simulink model "Eq_Zeq_circuit"  (R2022b)
settings: Solver=VariableStepAuto  StartTime=0.0  StopTime=10.0  RelTol=1e-3
libraries: nesl_utility x8, fl_lib x7, ee_lib x2
settings Model: Creator=umber  LastModifiedBy=umber

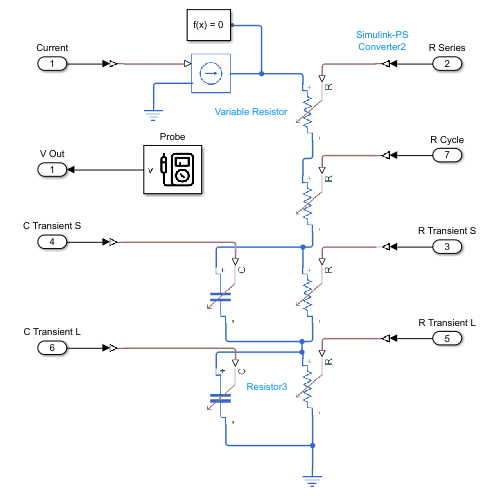
[thumbnail: Simulink's stored preview of the top-level diagram]
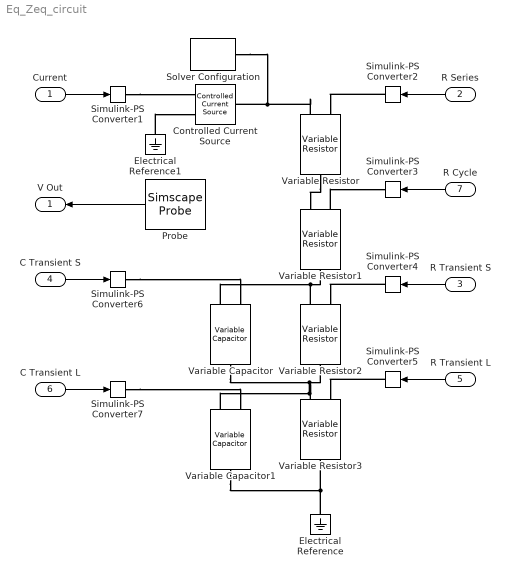
== system Eq_Zeq_circuit ==
  Current : Inport
  R Series : Inport  Port=2
  R Transient S : Inport  Port=3
  C Transient S : Inport  Port=4
  R Transient L : Inport  Port=5
  C Transient L : Inport  Port=6
  R Cycle : Inport  Port=7
  Controlled Current Source : fl_lib/Electrical/Electrical Sources/Controlled Current Source
  Electrical Reference : fl_lib/Electrical/Electrical Elements/Electrical Reference
  Electrical Reference1 : fl_lib/Electrical/Electrical Elements/Electrical Reference
  Probe : SimscapeProbe  BoundBlock=54  Variables={v}
  Simulink-PS Converter{1..7} (7 alike) : nesl_utility/Simulink-PS Converter  PhysicalDomain=network_engine_domain  SubClassName=ps_input  LeftPortType=input  RightPortType=output  PseudoPeriodic=off  Frequencies=[]  NoiseDistribution=none  NoiseParameters=[]  Unit=1  AffineConversion=off  FilteringAndDerivatives=provide  SimscapeFilterOrder=1  InputFilterTimeConstant=0.001  UdotUserProvided=0
  Solver Configuration : nesl_utility/Solver Configuration  PhysicalDomain=network_engine_domain  SubClassName=solver  LeftPortType=input  RightPortType=generic  Tones=[]  Harmonics=[]  SimulateNoise=off  Profile=off  UseLocalSampling=off  EnableSwitchedLinearOptims=on  FrequencyDomain=off  UseCCode=off  RelTol=0.001  AbsTol=0.001  MinStep=1e-09  ToWorkspace=off  RevertToSquareIcSolve=off  NumHomotopyIterations=100  PhasorMode=off  PhasorModeNumHarmonics=1  ConsistencySolver=NEWTON_XTOL_AFTER_FTOL  IndexReductionMethod=DerivativeReplacement  DoDC=off  ResidualTolerance=1e-09  ConsistencyTolSource=GLOBAL  ConsistencyAbsTol=0.001  ConsistencyRelTol=0.001  ConsistencyTolFactor=0.001  UseLocalSolver=off  LocalSolverChoice=NE_BACKWARD_EULER_ADVANCER  ResolveIndetEquations=on  FunctionEvalNumThread=1  LocalSolverSampleTime=0.001  DoFixedCost=off  MaxNonlinIter=3  MaxModeIter=2  ComputeImpulses=off  ImpulseIterations=2  LinearAlgebra=auto  LinearAlgebraNumThread=0  EquationFormulation=NE_TIME_EF  DelaysMemoryBudget=1024  AutomaticFiltering=on  FilteringTimeConstant=0.001  PartitionStorageMethod=AS_NEEDED  PartitionMemoryBudget=1024  PartitionMethod=ROBUST
  Variable Capacitor : ee_lib/Passive/Variable Capacitor  prm=2  Cmin=1e-9 F  r=1e-6 Ohm  v0=0 V  q0=0 C
      settings: InternalSimscapePortConfiguration="{\"Bottom\":[],\"Left\":[{\"id\":\"C\",\"label\":\"C\",\"type\":\"input\"},{\"id\":\"p\",\"label\":\"+\",\"type\":\"foundation.electrical.electrical\"}],\"Right\":[{\"id\":\"n\",\"label\":\"-\",\"type\":\"foundation.electrical.electrical\"}],\"Top\":[]}"
  Variable Capacitor1 : ee_lib/Passive/Variable Capacitor  prm=2  Cmin=1e-9 F  r=1e-6 Ohm  v0=0 V  q0=0 C
      settings: InternalSimscapePortConfiguration="{\"Bottom\":[],\"Left\":[{\"id\":\"C\",\"label\":\"C\",\"type\":\"input\"},{\"id\":\"p\",\"label\":\"+\",\"type\":\"foundation.electrical.electrical\"}],\"Right\":[{\"id\":\"n\",\"label\":\"-\",\"type\":\"foundation.electrical.electrical\"}],\"Top\":[]}"
  Variable Resistor{,1..3} (4 alike) : fl_lib/Electrical/Electrical Elements/Variable Resistor  Rmin=0 Ohm  i_specify=off  i_priority=None  i=0 A  i_nominal_specify=off  i_nominal_unit=A  i_nominal_value=1  v_specify=off  v_priority=None  v=0 V  v_nominal_specify=off  v_nominal_unit=V  v_nominal_value=1
  V Out : Outport
  wires:
  Current/1 -> Simulink-PS Converter1/1
  Probe/1 -> V Out/1
  R Series/1 -> Simulink-PS Converter2/1
  R Cycle/1 -> Simulink-PS Converter3/1
  R Transient S/1 -> Simulink-PS Converter4/1
  R Transient L/1 -> Simulink-PS Converter5/1
  C Transient S/1 -> Simulink-PS Converter6/1
  C Transient L/1 -> Simulink-PS Converter7/1
  connections:
  Simulink-PS Converter1/RConn1 -- Controlled Current Source/RConn1
  Electrical Reference1/LConn1 -- Controlled Current Source/RConn2
  Simulink-PS Converter2/RConn1 -- Variable Resistor/LConn1
  Variable Resistor1/LConn1 -- Simulink-PS Converter3/RConn1
  Simulink-PS Converter4/RConn1 -- Variable Resistor2/LConn1
  Simulink-PS Converter5/RConn1 -- Variable Resistor3/LConn1
  Variable Resistor2/LConn2 -- Variable Resistor1/RConn1 -- Variable Capacitor/LConn2
  Variable Resistor3/LConn2 -- Variable Capacitor1/LConn2 -- Variable Capacitor/RConn1 -- Variable Resistor2/RConn1
  Electrical Reference/LConn1 -- Variable Capacitor1/RConn1 -- Variable Resistor3/RConn1
  Variable Resistor/RConn1 -- Variable Resistor1/LConn2
  Variable Resistor/LConn2 -- Solver Configuration/RConn1 -- Controlled Current Source/LConn1
  Simulink-PS Converter7/RConn1 -- Variable Capacitor1/LConn1
  Simulink-PS Converter6/RConn1 -- Variable Capacitor/LConn1
